simulink model "TRAM"  (R2023b)
settings: Solver=VariableStepAuto  StartTime=0.0  StopTime=2000  MaxStep=1e-2  RelTol=1e-3
undefined symbols (not defined in the file): a_max, beta, E_n, J_eq, K_s, Ki_a, Ki_e, km_h_to_m_s, Kp_a, Kp_e, L_a, L_e, m_Total, overall_rated_current, pid_Mec, R_a, R_e, rated_i_excitation, rated_speed_rad_s, rated_v_excitation, rho, T_C_i_a, T_C_i_e, T_C_Mec, v_line, v_max, v_r_tram, w_dot_max, wheel_d
libraries: slpidlib x3
settings Model: Creator=felip  LastModifiedBy=franc
settings SolverCC: ZeroCrossAlgorithm=Adaptive  AlgebraicLoopSolver=TrustRegion
settings DebuggingCC: IgnoredZcDiagnostic=none
settings RTWCC: GPUComputeCapability=5.0  DLArmComputeVersion=19.05

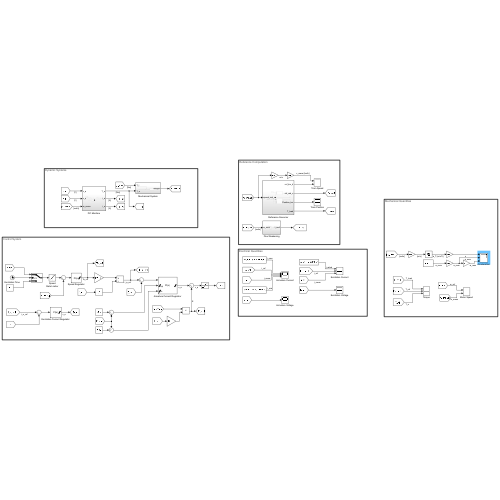
[thumbnail: Simulink's stored preview of the top-level diagram]
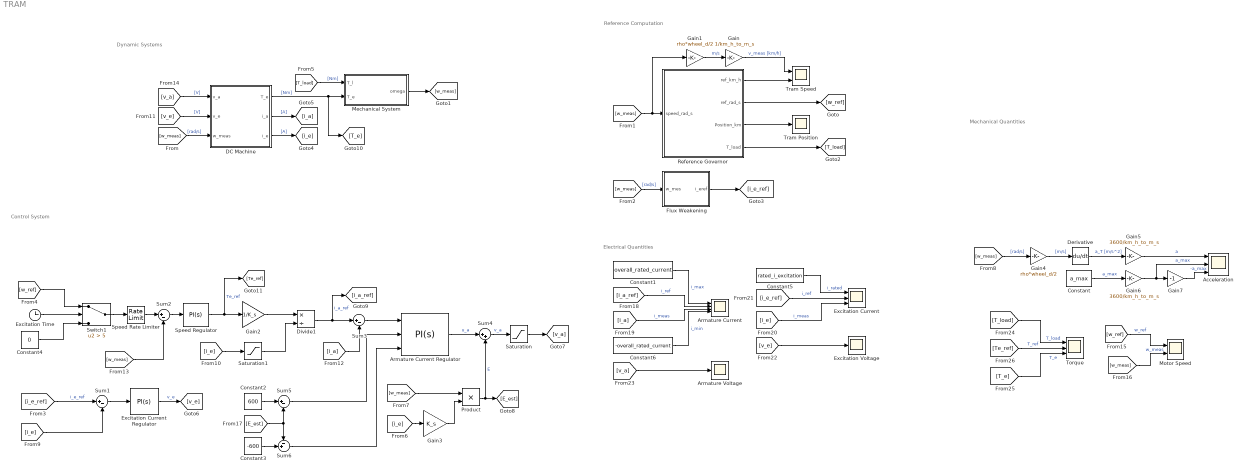
== system TRAM ==
  note: Dynamic Systems
  note: Mechanical Quantities
  note: Electrical Quantities
  note: Reference Computation
  note: Control System
  Acceleration : Scope  NumInputPorts=3
  Armature Current : Scope  NumInputPorts=4
  Armature Current Regulator : slpidlib/PID Controller  Controller=PI  Form=Parallel  TimeDomain=Continuous-time  UseExternalTs=off  SampleTime=-1  IntegratorMethod=Forward Euler  FilterMethod=Forward Euler  ControllerParametersSource=internal  P=Kp_a  I=Ki_a  UseKiTs=off  D=0  N=100  UseFilter=on  TunerSelectOption=Transfer Function Based (PID Tuner App)  ZeroCross=off  InitialConditionSource=internal  InitialConditionForIntegrator=0  InitialConditionForFilter=0  DifferentiatorICPrevScaledInput=0  ExternalReset=none  TrackingMode=off  Kt=1  LimitOutput=on  SatLimitsSource=external  UpperSaturationLimit=v_line  LowerSaturationLimit=-v_line  LinearizeAsGain=on  AntiWindupMode=clamping  Kb=1/T_C_i_a  LimitIntegrator=off  UpperIntegratorSaturationLimit=inf  LowerIntegratorSaturationLimit=-inf  POutMin=[]  POutMax=[]  IOutMin=[]  IOutMax=[]  DOutMin=[]  DOutMax=[]  NOutMin=[]  NOutMax=[]  SumOutMin=[]  SumOutMax=[]  SaturationOutMin=[]  SaturationOutMax=[]  PParamMin=[]  PParamMax=[]  IParamMin=[]  IParamMax=[]  DParamMin=[]  DParamMax=[]  NParamMin=[]  NParamMax=[]  KbParamMin=[]  KbParamMax=[]  KtParamMin=[]  KtParamMax=[]  KbOutMin=[]  KbOutMax=[]  KtOutMin=[]  KtOutMax=[]  IntegratorOutMin=[]  IntegratorOutMax=[]  FilterOutMin=[]  FilterOutMax=[]  SumI1OutMin=[]  SumI1OutMax=[]  SumI2OutMin=[]  SumI2OutMax=[]  SumI3OutMin=[]  SumI3OutMax=[]  SumI4OutMin=[]  SumI4OutMax=[]  SumDOutMin=[]  SumDOutMax=[]  DifferentiatorOutMin=[]  DifferentiatorOutMax=[]  FilterDiffOutCoefMin=[]  FilterDiffOutCoefMax=[]  ReciprocalOutMin=[]  ReciprocalOutMax=[]  SumDenOutMin=[]  SumDenOutMax=[]  SumNumOutMin=[]  SumNumOutMax=[]  DivideOutMin=[]  DivideOutMax=[]  UdiffTsProdOutMin=[]  UdiffTsProdOutMax=[]  NTsProdOutMin=[]  NTsProdOutMax=[]  UintegralTsProdOutMin=[]  UintegralTsProdOutMax=[]  UngainTsProdOutMin=[]  UngainTsProdOutMax=[]  ClampingZeroOutDataTypeStr=Inherit: Inherit via back propagation  ClampingZeroOutMin=[]  ClampingZeroOutMax=[]  FilterDenConstantOutDataTypeStr=Inherit: Inherit via back propagation  FilterDenConstantOutMin=[]  FilterDenConstantOutMax=[]  PCopyOutDataTypeStr=Inherit: Inherit via back propagation  PCopyOutMin=[]  PCopyOutMax=[]  NCopyOutDataTypeStr=Inherit: Inherit via back propagation  NCopyOutMin=[]  NCopyOutMax=[]  IntegratorContinuousStateAttributes=''  IntegratorStateMustResolveToSignalObject=off  IntegratorRTWStateStorageClass=Auto  FilterContinuousStateAttributes=''  FilterStateMustResolveToSignalObject=off  FilterRTWStateStorageClass=Auto  ParallelPVariant=InternalParameters  IdealPVariant=Disabled  IVariant=InternalParameters  DVariant=Disabled  IntegratorVariant=Continuous  SatVariant=External  AWVariant=ContClampingParallel  PCopyVariant=Disabled  TRVariant=Disabled  FdbkBlocksVariant=Forward  IdealPFdbkVariant=Disabled  SatFdbkVariant=Disabled  DerivativeFilterVariant=Disabled  NVariant=Disabled  NCopyVariant=Disabled_SignalSpec  FilterICVariant=Disabled  IntegratorICVariant=InternalICs  ExternalResetVariant=Disabled  TRSumVariant=Passthrough  SumFdbkVariant=Disabled  SumVariant=Sum_PI  TsampFilterVariant=InternalTs  TsampNgainVariant=Passthrough  TsampIntegralVariant=Disabled_SignalSpec  ExternalSaturationOutDataTypeStr=Inherit: Same as second input
  Armature Voltage : Scope
  Constant : Constant  Value=a_max
  Constant1 : Constant  Value=overall_rated_current
  Constant2 : Constant  Value=600
  Constant3 : Constant  Value=-600
  Constant4 : Constant  Value=0
  Constant5 : Constant  Value=rated_i_excitation
  Constant6 : Constant  Value=-overall_rated_current
  DC Machine : Subsystem
  Derivative : Derivative
  Divide1 : Product  Inputs=*/
  Excitation Current : Scope  NumInputPorts=3
  Excitation Current Regulator : slpidlib/PID Controller  Controller=PI  Form=Parallel  TimeDomain=Continuous-time  UseExternalTs=off  SampleTime=-1  IntegratorMethod=Forward Euler  FilterMethod=Forward Euler  ControllerParametersSource=internal  P=Kp_e  I=Ki_e  UseKiTs=off  D=0  N=100  UseFilter=on  TunerSelectOption=Transfer Function Based (PID Tuner App)  ZeroCross=off  InitialConditionSource=internal  InitialConditionForIntegrator=0  InitialConditionForFilter=0  DifferentiatorICPrevScaledInput=0  ExternalReset=none  TrackingMode=off  Kt=1  LimitOutput=on  SatLimitsSource=internal  UpperSaturationLimit=rated_v_excitation  LowerSaturationLimit=-rated_v_excitation  LinearizeAsGain=on  AntiWindupMode=clamping  Kb=1/T_C_i_e  LimitIntegrator=off  UpperIntegratorSaturationLimit=inf  LowerIntegratorSaturationLimit=-inf  POutMin=[]  POutMax=[]  IOutMin=[]  IOutMax=[]  DOutMin=[]  DOutMax=[]  NOutMin=[]  NOutMax=[]  SumOutMin=[]  SumOutMax=[]  SaturationOutMin=[]  SaturationOutMax=[]  PParamMin=[]  PParamMax=[]  IParamMin=[]  IParamMax=[]  DParamMin=[]  DParamMax=[]  NParamMin=[]  NParamMax=[]  KbParamMin=[]  KbParamMax=[]  KtParamMin=[]  KtParamMax=[]  KbOutMin=[]  KbOutMax=[]  KtOutMin=[]  KtOutMax=[]  IntegratorOutMin=[]  IntegratorOutMax=[]  FilterOutMin=[]  FilterOutMax=[]  SumI1OutMin=[]  SumI1OutMax=[]  SumI2OutMin=[]  SumI2OutMax=[]  SumI3OutMin=[]  SumI3OutMax=[]  SumI4OutMin=[]  SumI4OutMax=[]  SumDOutMin=[]  SumDOutMax=[]  DifferentiatorOutMin=[]  DifferentiatorOutMax=[]  FilterDiffOutCoefMin=[]  FilterDiffOutCoefMax=[]  ReciprocalOutMin=[]  ReciprocalOutMax=[]  SumDenOutMin=[]  SumDenOutMax=[]  SumNumOutMin=[]  SumNumOutMax=[]  DivideOutMin=[]  DivideOutMax=[]  UdiffTsProdOutMin=[]  UdiffTsProdOutMax=[]  NTsProdOutMin=[]  NTsProdOutMax=[]  UintegralTsProdOutMin=[]  UintegralTsProdOutMax=[]  UngainTsProdOutMin=[]  UngainTsProdOutMax=[]  ClampingZeroOutDataTypeStr=Inherit: Inherit via back propagation  ClampingZeroOutMin=[]  ClampingZeroOutMax=[]  FilterDenConstantOutDataTypeStr=Inherit: Inherit via back propagation  FilterDenConstantOutMin=[]  FilterDenConstantOutMax=[]  PCopyOutDataTypeStr=Inherit: Inherit via back propagation  PCopyOutMin=[]  PCopyOutMax=[]  NCopyOutDataTypeStr=Inherit: Inherit via back propagation  NCopyOutMin=[]  NCopyOutMax=[]  IntegratorContinuousStateAttributes=''  IntegratorStateMustResolveToSignalObject=off  IntegratorRTWStateStorageClass=Auto  FilterContinuousStateAttributes=''  FilterStateMustResolveToSignalObject=off  FilterRTWStateStorageClass=Auto  ParallelPVariant=InternalParameters  IdealPVariant=Disabled  IVariant=InternalParameters  DVariant=Disabled  IntegratorVariant=Continuous  SatVariant=Enabled  AWVariant=ContClampingParallel  PCopyVariant=Disabled  TRVariant=Disabled  FdbkBlocksVariant=Forward  IdealPFdbkVariant=Disabled  SatFdbkVariant=Disabled  DerivativeFilterVariant=Disabled  NVariant=Disabled  NCopyVariant=Disabled_SignalSpec  FilterICVariant=Disabled  IntegratorICVariant=InternalICs  ExternalResetVariant=Disabled  TRSumVariant=Passthrough  SumFdbkVariant=Disabled  SumVariant=Sum_PI  TsampFilterVariant=InternalTs  TsampNgainVariant=Passthrough  TsampIntegralVariant=Disabled_SignalSpec  ExternalSaturationOutDataTypeStr=Inherit: Same as second input
  Excitation Time : Clock
  Excitation Voltage : Scope
  Flux Weakening : Subsystem
  Gain : Gain  Gain=1/km_h_to_m_s
  Gain1 : Gain  Gain=rho*wheel_d/2
  Gain2 : Gain  Gain=1/K_s
  Gain3 : Gain  Gain=K_s
  Gain4 : Gain  Gain=rho*wheel_d/2
  Gain5 : Gain  Gain=3600/km_h_to_m_s
  Gain6 : Gain  Gain=3600/km_h_to_m_s
  Gain7 : Gain  Gain=-1
  Mechanical System : Subsystem
  Motor Speed : Scope  NumInputPorts=2
  Product : Product
  Reference Governor : Subsystem
  Saturation : Saturate  UpperLimit=v_line  LowerLimit=-v_line  ZeroCross=off
  Saturation1 : Saturate  UpperLimit=inf  LowerLimit=1
  Speed Rate Limiter : RateLimiter  RisingSlewLimit=w_dot_max  FallingSlewLimit=-w_dot_max  SampleTimeMode=inherited
  Speed Regulator : slpidlib/PID Controller  Controller=PI  Form=Parallel  TimeDomain=Continuous-time  UseExternalTs=off  SampleTime=-1  IntegratorMethod=Forward Euler  FilterMethod=Forward Euler  ControllerParametersSource=internal  P=93  I=7  UseKiTs=off  D=pid_Mec.Kd  N=100  UseFilter=on  TunerSelectOption=Transfer Function Based (PID Tuner App)  ZeroCross=off  InitialConditionSource=internal  InitialConditionForIntegrator=0  InitialConditionForFilter=0  DifferentiatorICPrevScaledInput=0  ExternalReset=none  TrackingMode=off  Kt=1  LimitOutput=on  SatLimitsSource=internal  UpperSaturationLimit=inf  LowerSaturationLimit=-inf  LinearizeAsGain=on  AntiWindupMode=clamping  Kb=1/T_C_Mec  LimitIntegrator=off  UpperIntegratorSaturationLimit=inf  LowerIntegratorSaturationLimit=-inf  POutMin=[]  POutMax=[]  IOutMin=[]  IOutMax=[]  DOutMin=[]  DOutMax=[]  NOutMin=[]  NOutMax=[]  SumOutMin=[]  SumOutMax=[]  SaturationOutMin=[]  SaturationOutMax=[]  PParamMin=[]  PParamMax=[]  IParamMin=[]  IParamMax=[]  DParamMin=[]  DParamMax=[]  NParamMin=[]  NParamMax=[]  KbParamMin=[]  KbParamMax=[]  KtParamMin=[]  KtParamMax=[]  KbOutMin=[]  KbOutMax=[]  KtOutMin=[]  KtOutMax=[]  IntegratorOutMin=[]  IntegratorOutMax=[]  FilterOutMin=[]  FilterOutMax=[]  SumI1OutMin=[]  SumI1OutMax=[]  SumI2OutMin=[]  SumI2OutMax=[]  SumI3OutMin=[]  SumI3OutMax=[]  SumI4OutMin=[]  SumI4OutMax=[]  SumDOutMin=[]  SumDOutMax=[]  DifferentiatorOutMin=[]  DifferentiatorOutMax=[]  FilterDiffOutCoefMin=[]  FilterDiffOutCoefMax=[]  ReciprocalOutMin=[]  ReciprocalOutMax=[]  SumDenOutMin=[]  SumDenOutMax=[]  SumNumOutMin=[]  SumNumOutMax=[]  DivideOutMin=[]  DivideOutMax=[]  UdiffTsProdOutMin=[]  UdiffTsProdOutMax=[]  NTsProdOutMin=[]  NTsProdOutMax=[]  UintegralTsProdOutMin=[]  UintegralTsProdOutMax=[]  UngainTsProdOutMin=[]  UngainTsProdOutMax=[]  ClampingZeroOutDataTypeStr=Inherit: Inherit via back propagation  ClampingZeroOutMin=[]  ClampingZeroOutMax=[]  FilterDenConstantOutDataTypeStr=Inherit: Inherit via back propagation  FilterDenConstantOutMin=[]  FilterDenConstantOutMax=[]  PCopyOutDataTypeStr=Inherit: Inherit via back propagation  PCopyOutMin=[]  PCopyOutMax=[]  NCopyOutDataTypeStr=Inherit: Inherit via back propagation  NCopyOutMin=[]  NCopyOutMax=[]  IntegratorContinuousStateAttributes=''  IntegratorStateMustResolveToSignalObject=off  IntegratorRTWStateStorageClass=Auto  FilterContinuousStateAttributes=''  FilterStateMustResolveToSignalObject=off  FilterRTWStateStorageClass=Auto  ParallelPVariant=InternalParameters  IdealPVariant=Disabled  IVariant=InternalParameters  DVariant=Disabled  IntegratorVariant=Continuous  SatVariant=Enabled  AWVariant=ContClampingParallel  PCopyVariant=Disabled  TRVariant=Disabled  FdbkBlocksVariant=Forward  IdealPFdbkVariant=Disabled  SatFdbkVariant=Disabled  DerivativeFilterVariant=Disabled  NVariant=Disabled  NCopyVariant=Disabled_SignalSpec  FilterICVariant=Disabled  IntegratorICVariant=InternalICs  ExternalResetVariant=Disabled  TRSumVariant=Passthrough  SumFdbkVariant=Disabled  SumVariant=Sum_PI  TsampFilterVariant=InternalTs  TsampNgainVariant=Passthrough  TsampIntegralVariant=Disabled_SignalSpec  ExternalSaturationOutDataTypeStr=Inherit: Same as second input
  Sum{1..3,5} (4 alike) : Sum  Inputs=|+-
  Sum4 : Sum  Inputs=|++
  Sum6 : Sum  Inputs=-+|
  Switch1 : Switch  Criteria=u2 > Threshold  Threshold=5  SaturateOnIntegerOverflow=off  InputSameDT=off
  Torque : Scope  NumInputPorts=3
  Tram Position : Scope
  Tram Speed : Scope  NumInputPorts=2
  wires:
  Reference Governor/1(ref_km_h) -> Tram Speed/2
  Reference Governor/2(ref_rad_s) -> [w_ref]
  [w_meas] -> Gain1/1, Reference Governor/1(speed_rad_s)
  Reference Governor/4(T_load) -> [T_load]
  Reference Governor/3(Position_km) -> Tram Position/1
  [i_e_ref] -> Sum1/1  "i_e_ref"
  Sum1/1 -> Excitation Current Regulator/1
  Sum3/1 -> Armature Current Regulator/1
  [i_e] -> Gain3/1
  Gain3/1 -> Product/2
  [w_meas] -> Product/1
  Gain4/1 -> Derivative/1  "[m/s]"
  [w_meas] -> Gain4/1  "[rad/s]"
  Derivative/1 -> Gain5/1  "a_T [m/s^2]"
  Constant/1 -> Gain6/1  "a_max"
  Gain2/1 -> Divide1/1
  Saturation1/1 -> Divide1/2
  [i_e] -> Saturation1/1
  Gain5/1 -> Acceleration/1  "a"
  Gain6/1 -> Acceleration/2, Gain7/1  "a_max"
  Gain7/1 -> Acceleration/3  "-a_max"
  Divide1/1 -> [i_a_ref], Sum3/1  "i_a_ref"
  Excitation Time/1 -> Switch1/2
  Constant4/1 -> Switch1/3
  [w_ref] -> Switch1/1
  DC Machine/3(i_e) -> [i_e]  "[A]"
  DC Machine/2(i_a) -> [i_a]  "[A]"
  [w_meas] -> DC Machine/3(w_meas)  "[rad/s]"
  [T_load] -> Mechanical System/1(T_l)  "[Nm]"
  DC Machine/1(T_e) -> [T_e], Mechanical System/2(T_e)  "[Nm]"
  Mechanical System/1(omega) -> [w_meas]
  Excitation Current Regulator/1 -> [v_e]  "v_e"
  [i_e] -> Sum1/2
  [v_e] -> DC Machine/2(v_e)  "[V]"
  [i_a] -> Sum3/2
  [w_meas] -> Sum2/2
  [w_meas] -> Flux Weakening/1(w_mes)  "[rad/s]"
  Flux Weakening/1(i_eref) -> [i_e_ref]
  [v_a] -> DC Machine/1(v_a)  "[V]"
  [w_ref] -> Motor Speed/1  "w_ref"
  [w_meas] -> Motor Speed/2  "w_meas"
  Gain1/1 -> Gain/1  "m/s"
  Gain/1 -> Tram Speed/1  "v_meas [km/h]"
  Sum4/1 -> Saturation/1  "v_a"
  Saturation/1 -> [v_a]
  Speed Regulator/1 -> [Te_ref], Gain2/1  "Te_ref"
  Product/1 -> [E_est], Sum4/2  "E"
  Sum6/1 -> Armature Current Regulator/3
  Sum5/1 -> Armature Current Regulator/2
  [i_a_ref] -> Armature Current/2  "i_ref"
  [i_a] -> Armature Current/3  "i_meas"
  Constant1/1 -> Armature Current/1  "i_max"
  Constant5/1 -> Excitation Current/1  "i_rated"
  [i_e_ref] -> Excitation Current/2  "i_ref"
  [i_e] -> Excitation Current/3  "i_meas"
  [v_e] -> Excitation Voltage/1
  [v_a] -> Armature Voltage/1
  [T_load] -> Torque/1  "T_load"
  [Te_ref] -> Torque/2  "T_ref"
  [T_e] -> Torque/3  "T_e"
  Sum2/1 -> Speed Regulator/1
  Switch1/1 -> Speed Rate Limiter/1
  Speed Rate Limiter/1 -> Sum2/1
  Constant6/1 -> Armature Current/4  "i_min"
  Armature Current Regulator/1 -> Sum4/1  "u_a"
  Constant2/1 -> Sum5/1
  Constant3/1 -> Sum6/2
  [E_est] -> Sum6/1, Sum5/2

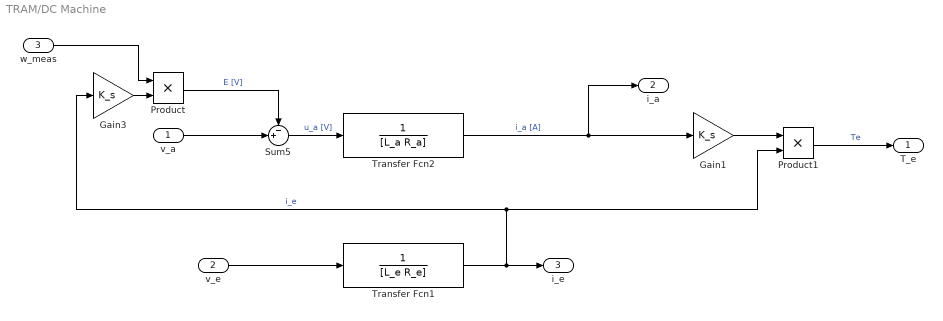
== system TRAM/DC Machine ==
  v_a : Inport
  v_e : Inport  Port=2
  w_meas : Inport  Port=3
  Gain1 : Gain  Gain=K_s
  Gain3 : Gain  Gain=K_s
  Product : Product
  Product1 : Product
  Sum5 : Sum  Inputs=-+|
  Transfer Fcn1 : TransferFcn  Denominator=[L_e R_e]
  Transfer Fcn2 : TransferFcn  Denominator=[L_a R_a]
  T_e : Outport
  i_a : Outport  Port=2
  i_e : Outport  Port=3
  wires:
  Gain1/1 -> Product1/1
  Sum5/1 -> Transfer Fcn2/1  "u_a [V]"
  Transfer Fcn1/1 -> Gain3/1, Product1/2, i_e/1  "i_e"
  Transfer Fcn2/1 -> i_a/1, Gain1/1  "i_a [A]"
  Product1/1 -> T_e/1  "Te"
  v_e/1 -> Transfer Fcn1/1
  v_a/1 -> Sum5/2
  Gain3/1 -> Product/2
  Product/1 -> Sum5/1  "E [V]"
  w_meas/1 -> Product/1

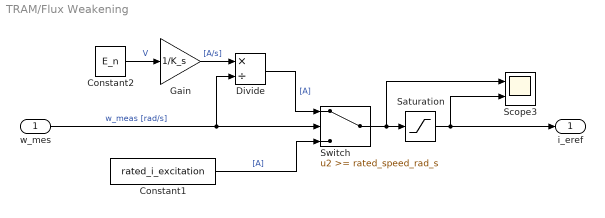
== system TRAM/Flux Weakening ==
  w_mes : Inport
  Constant1 : Constant  Value=rated_i_excitation
  Constant2 : Constant  Value=E_n
  Divide : Product  Inputs=*/
  Gain : Gain  Gain=1/K_s
  Saturation : Saturate  UpperLimit=rated_i_excitation  LowerLimit=-rated_i_excitation
  Scope3 : Scope  NumInputPorts=2
  Switch : Switch  Threshold=rated_speed_rad_s  SaturateOnIntegerOverflow=off  InputSameDT=off
  i_eref : Outport
  wires:
  w_mes/1 -> Divide/2, Switch/2  "w_meas [rad/s]"
  Gain/1 -> Divide/1  "[A/s]"
  Switch/1 -> Scope3/1, Saturation/1
  Constant1/1 -> Switch/3  "[A]"
  Constant2/1 -> Gain/1  "V"
  Divide/1 -> Switch/1  "[A]"
  Saturation/1 -> i_eref/1, Scope3/2

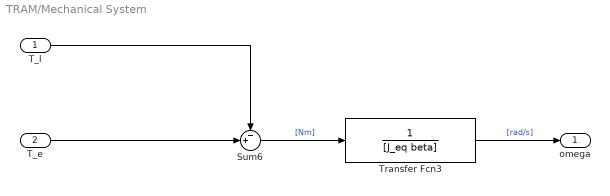
== system TRAM/Mechanical System ==
  T_l : Inport
  T_e : Inport  Port=2
  Sum6 : Sum  Inputs=-+|
  Transfer Fcn3 : TransferFcn  Denominator=[J_eq beta]
  omega : Outport
  wires:
  T_e/1 -> Sum6/2
  Sum6/1 -> Transfer Fcn3/1  "[Nm]"
  Transfer Fcn3/1 -> omega/1  "[rad/s]"
  T_l/1 -> Sum6/1

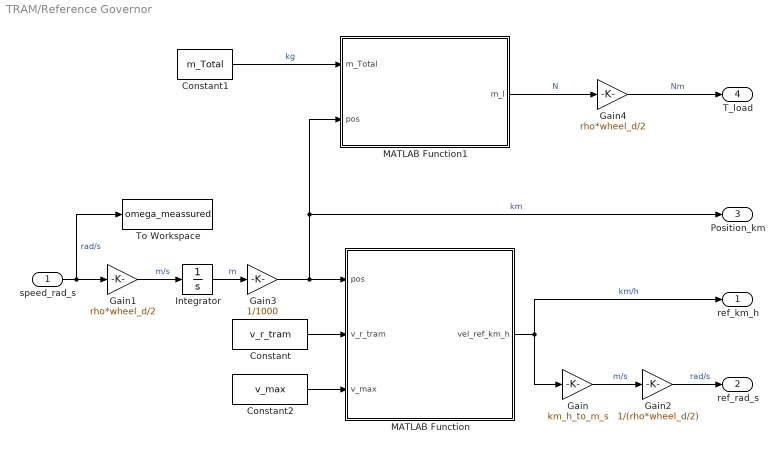
== system TRAM/Reference Governor ==
  speed_rad_s : Inport
  Constant : Constant  Value=v_r_tram
  Constant1 : Constant  Value=m_Total
  Constant2 : Constant  Value=v_max
  Gain : Gain  Gain=km_h_to_m_s
  Gain1 : Gain  Gain=rho*wheel_d/2
  Gain2 : Gain  Gain=1/(rho*wheel_d/2)
  Gain3 : Gain  Gain=1/1000
  Gain4 : Gain  Gain=rho*wheel_d/2
  Integrator : Integrator
  MATLAB Function : MATLAB Function  TreatAsAtomicUnit=on
  MATLAB Function1 : MATLAB Function  TreatAsAtomicUnit=on
  To Workspace : ToWorkspace  VariableName=omega_meassured  SaveFormat=Timeseries  SampleTime=-1
  ref_km_h : Outport
  ref_rad_s : Outport  Port=2
  Position_km : Outport  Port=3
  T_load : Outport  Port=4
  wires:
  Gain1/1 -> Integrator/1  "m/s"
  Integrator/1 -> Gain3/1  "m"
  Constant/1 -> MATLAB Function/2(v_r_tram)
  Constant2/1 -> MATLAB Function/3(v_max)
  MATLAB Function/1(vel_ref_km_h) -> ref_km_h/1, Gain/1  "km/h"
  speed_rad_s/1 -> To Workspace/1, Gain1/1  "rad/s"
  Gain2/1 -> ref_rad_s/1  "rad/s"
  Gain/1 -> Gain2/1  "m/s"
  Gain3/1 -> MATLAB Function1/2(pos), Position_km/1, MATLAB Function/1(pos)  "km"
  Constant1/1 -> MATLAB Function1/1(m_Total)  "kg"
  MATLAB Function1/1(m_l) -> Gain4/1  "N"
  Gain4/1 -> T_load/1  "Nm"

== matlab function TRAM/Reference Governor/MATLAB Function1 ==
  data: m_Total input; pos input; m_l output
function m_l  = tram_slip_profile(m_Total, pos)

    m_l = (m_Total*9.81*sin(atan(5/100)))*(1.*step(pos-3) + ...
               -1.*step(pos-4) - ...
                1.*step(pos-8) + ...
                1.*step(pos-9));
end

function y = step(t)
    y = 1.*(t>0);
end

== matlab function TRAM/Reference Governor/MATLAB Function ==
  data: pos input; vel_ref_km_h output; v_r_tram input; v_max input
function vel_ref_km_h  = tram_vel_profile(pos, v_r_tram, v_max)

    vel_ref_km_h = v_r_tram/2+ ...
               v_r_tram/2.*step_u(pos-1) + ...
               (v_max-v_r_tram).*step_u(pos-4) - ...
               (v_max-v_r_tram).*step_u(pos-6) - ...
               v_r_tram/2.*step_u(pos-9) - ...
               v_r_tram/2.*step_u(pos-10);
end

function y = step_u(t)
    y = 1.*(t>0);
end
